simulink model "A02_L07_1"  (R2021b)
settings: Solver=ode45  StartTime=0.0  StopTime=100  RelTol=1e-3
undefined symbols (not defined in the file or in its folder): Ki, Kp
settings Model: Creator=User  LastModifiedBy=mluser
settings SolverCC: AlgebraicLoopSolver=TrustRegion
settings DataIOCC: LimitDataPoints=on  SaveFormat=Array  ReturnWorkspaceOutputs=off
settings OptimizationCC: BlockReduction=off  BooleanDataType=off  LifeSpan=inf
settings DebuggingCC: SaveWithParameterizedLinksMsg=none  UnderspecifiedInitializationDetection=Classic  MergeDetectMultiDrivingBlocksExec=none  SignalResolutionControl=TryResolveAllWithWarning  SFUnexpectedBacktrackingDiag=warning  SFNoUnconditionalDefaultTransitionDiag=warning  SFExecutionAtInitializationDiag=none  SFMachineParentedDataDiag=warning  ArithmeticOperatorsInVariantConditions=warning
settings HardwareCC: ProdBitPerPointer=32  ProdBitPerSizeT=32  ProdBitPerPtrDiffT=32  ProdLargestAtomicFloat=None  ProdIntDivRoundTo=Undefined  ProdEndianess=Unspecified  ProdWordSize=32  ProdHWDeviceType=32-bit Generic  TargetUnknown=on
settings ModelReferenceCC: PropagateSignalLabelsOutOfModel=off
settings SFSimCC: SimUseLocalCustomCode=off  CustomCodeUndefinedFunction=UseInterfaceOnly
settings RTWCC: RTWUseLocalCustomCode=off
settings CodeAppCC: StateflowObjectComments=on
settings GRTTargetCC: TargetLangStandard=C89/C90 (ANSI)
settings ConfigComp: CovMetricSettings=dw  CovSaveCumulativeToWorkspaceVar=on  CovSaveSingleToWorkspaceVar=on  CovExternalEMLEnable=off  CovSFcnEnable=off

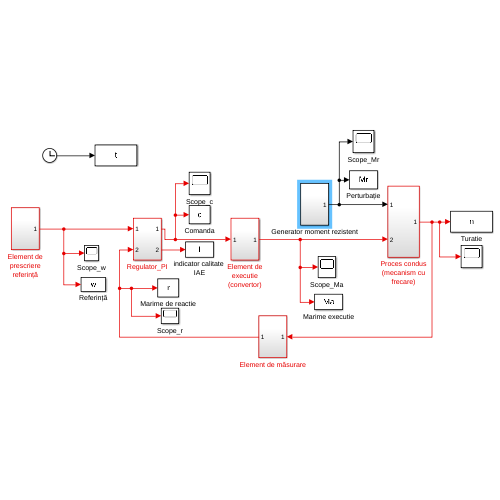
[thumbnail: Simulink's stored preview of the top-level diagram]
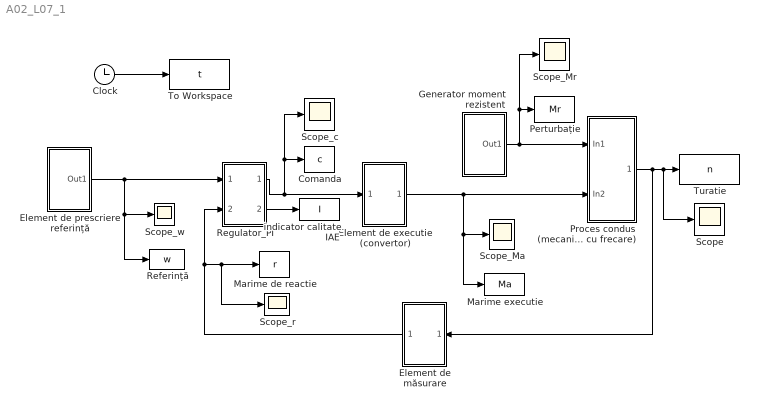
== system A02_L07_1 ==
  Clock : Clock
  Comanda : ToWorkspace  VariableName=c  SampleTime=-1
  Element de executie (convertor) : Subsystem
  Element de prescriere referință : Subsystem
  Element de măsurare : Subsystem
  Generator moment rezistent : Subsystem
  Marime de reactie : ToWorkspace  VariableName=r  SampleTime=-1
  Marime executie : ToWorkspace  VariableName=Ma  SampleTime=-1
  Perturbație : ToWorkspace  VariableName=Mr  SampleTime=-1
  Proces condus (mecanism cu frecare) : Subsystem
  Referință : ToWorkspace  VariableName=w  SampleTime=-1
  Regulator_PI : Subsystem
  Scope : Scope
  Scope_Ma : Scope
  Scope_Mr : Scope
  Scope_c : Scope
  Scope_r : Scope
  Scope_w : Scope
  To Workspace : ToWorkspace  VariableName=t  SampleTime=-1
  Turatie : ToWorkspace  VariableName=n  SampleTime=-1
  indicator calitate IAE : ToWorkspace  VariableName=I  SampleTime=-1
  wires:
  Clock/1 -> To Workspace/1
  Proces condus (mecanism cu frecare)/1(Out1) -> Element de măsurare/1(In1), Scope/1, Turatie/1
  Regulator_PI/1(Out1) -> Element de executie (convertor)/1(In1), Scope_c/1, Comanda/1
  Element de prescriere referință/1(Out1) -> Scope_w/1, Referință/1, Regulator_PI/1(In1)
  Generator moment rezistent/1(Out1) -> Proces condus (mecanism cu frecare)/1(In1), Scope_Mr/1, Perturbație/1
  Element de executie (convertor)/1(Out1) -> Scope_Ma/1, Marime executie/1, Proces condus (mecanism cu frecare)/2(In2)
  Element de măsurare/1(Out1) -> Scope_r/1, Marime de reactie/1, Regulator_PI/2(In2)
  Regulator_PI/2(Out2) -> indicator calitate IAE/1

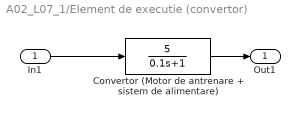
== system A02_L07_1/Element de executie (convertor) ==
  In1 : Inport
  Convertor (Motor de antrenare + sistem de alimentare) : TransferFcn  Numerator=[5]  Denominator=[0.1 1]
  Out1 : Outport  VectorParamsAs1DForOutWhenUnconnected=off
  wires:
  In1/1 -> Convertor (Motor de antrenare + sistem de alimentare)/1
  Convertor (Motor de antrenare + sistem de alimentare)/1 -> Out1/1

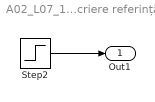
== system A02_L07_1/Element de prescriere referință ==
  Step2 : Step  Time=0  After=15  SampleTime=0
  Out1 : Outport  VectorParamsAs1DForOutWhenUnconnected=off
  wires:
  Step2/1 -> Out1/1

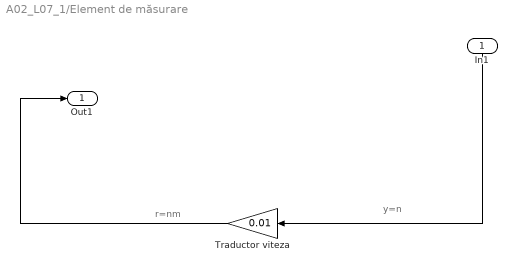
== system A02_L07_1/Element de măsurare ==
  note: r=nm
  note: y=n
  In1 : Inport
  Traductor viteza : Gain  Gain=0.01
  Out1 : Outport  VectorParamsAs1DForOutWhenUnconnected=off
  wires:
  In1/1 -> Traductor viteza/1
  Traductor viteza/1 -> Out1/1

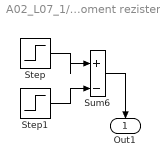
== system A02_L07_1/Generator moment rezistent ==
  Step : Step  Time=55  After=50  SampleTime=0
  Step1 : Step  Time=65  After=50  SampleTime=0
  Sum6 : Sum  Inputs=|+-
  Out1 : Outport  VectorParamsAs1DForOutWhenUnconnected=off
  wires:
  Sum6/1 -> Out1/1
  Step/1 -> Sum6/1
  Step1/1 -> Sum6/2

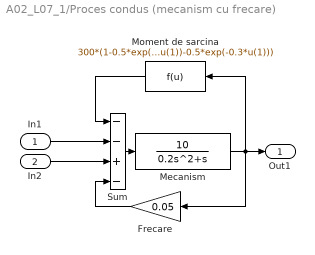
== system A02_L07_1/Proces condus (mecanism cu frecare) ==
  In1 : Inport
  In2 : Inport  Port=2
  Frecare : Gain  Gain=0.05
  Mecanism : TransferFcn  Numerator=[10]  Denominator=[0.2 1 0]
  Moment de sarcina : Fcn  Expr=300*(1-0.5*exp(-u(1))-0.5*exp(-0.3*u(1)))
  Sum : Sum  Inputs=--+-
  Out1 : Outport  VectorParamsAs1DForOutWhenUnconnected=off
  wires:
  Sum/1 -> Mecanism/1
  Mecanism/1 -> Out1/1, Moment de sarcina/1, Frecare/1
  Frecare/1 -> Sum/4
  In2/1 -> Sum/3
  In1/1 -> Sum/2
  Moment de sarcina/1 -> Sum/1

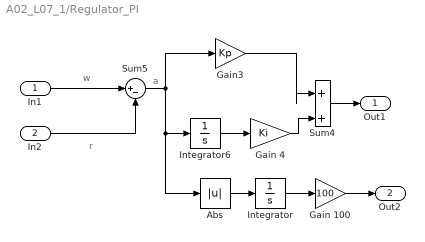
== system A02_L07_1/Regulator_PI ==
  note: a
  note: r
  note: w
  In1 : Inport
  In2 : Inport  Port=2
  Abs : Abs
  Gain 100 : Gain  Gain=100
  Gain 4 : Gain  Gain=Ki
  Gain3 : Gain  Gain=Kp
  Integrator : Integrator
  Integrator6 : Integrator
  Sum4 : Sum  Inputs=|++
  Sum5 : Sum  Inputs=|+-
  Out1 : Outport  VectorParamsAs1DForOutWhenUnconnected=off
  Out2 : Outport  Port=2  VectorParamsAs1DForOutWhenUnconnected=off
  wires:
  Sum5/1 -> Abs/1, Integrator6/1, Gain3/1
  Integrator6/1 -> Gain 4/1
  In2/1 -> Sum5/2
  Sum4/1 -> Out1/1
  Gain3/1 -> Sum4/1
  In1/1 -> Sum5/1
  Gain 4/1 -> Sum4/2
  Abs/1 -> Integrator/1
  Integrator/1 -> Gain 100/1
  Gain 100/1 -> Out2/1
